simulink library "arduinodue_drivers"  (R2015a)
settings: Solver=ode45  StartTime=0.0  StopTime=10.0  FixedStep=0.01  RelTol=1e-3
settings Model: CovSFcnEnable=off  Creator=odufour  LastModifiedBy=tbaroche
settings DataIOCC: LimitDataPoints=off  SignalLoggingSaveFormat=ModelDataLogs  SignalLogging=off  DSMLogging=off
settings DebuggingCC: UnderspecifiedInitializationDetection=Classic  MergeDetectMultiDrivingBlocksExec=none  SolverPrmCheckMsg=warning
settings GRTTargetCC: CombineOutputUpdateFcns=off  GRTInterface=on

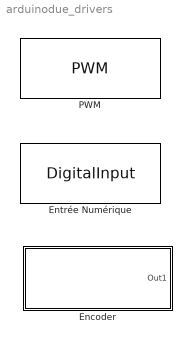
== system arduinodue_drivers ==
  Encoder : Subsystem  mask{pinA=18, pinB=19}
      mask prompts: pinA "Pin A"; pinB "Pin B"
      mask help:
      | Se bloc permet de récupérer le nombre d'incrément qui ont été effectué depuis le lancement de la simulation. Les changements de sens de rotation éventuels sont pris en compte. Ceci permet alors de pouvoir estimer la distance parcourrue.
      |
      | Il est nécessaire d'indiquer les deux entrées sur lesquels est connecté l'encodeur.
      mask Display: disp('Arduino Encoder')
  Entrée Numérique : S-Function  FunctionName=DigitalInput  Parameters=pinNumber, isPullUp  mask(Arduino Digital Input){pinNumber=0, isPullUp=on}
      mask prompts: pinNumber "Pin Number"; isPullUp "Enable Pull Up"
      mask help:
      | Get the logical value of a specified digital input pin.
      |
      | Enter the number of the digital input pin (0-53 for Arduino Due). Do not assign the same pin number to multiple blocks within a model.
      mask init:
      | % Make sure that data type of pinNumber is UINT8
      | pinNumber = uint8(pinNumber);
      | 
      | % Make sure that data type of isPullUp is UINT8
      | isPullUp = uint8(isPullUp);
      mask Display: disp(sprintf('Arduino Digital Input\nPin n°%d',pinNumber))
  PWM : S-Function  FunctionName=PWM  Parameters=pinNumber  mask(Arduino PWM){pinNumber=2}
      mask prompts: pinNumber "Pin Number"
      mask help:
      | Generate square waveform on the specified analog output pin. The block input controls the duty cycle of the square waveform. An input value of 0 produces a 0 percent duty cycle, and an input value of 255 produces a 100 percent duty cycle. The frequency of the waveform is constant at approximately 490 Hz.
      |
      | Enter the number of the analog output pin (2-13 for Arduino Due). Do not assign the same pin number to multiple blocks within a model.
      mask init:
      | % Make sure that pinNumber is an INT32
      | pinNumber = int32(pinNumber);
      mask Display: disp(sprintf('Arduino PWM\nPin n°%d',pinNumber))

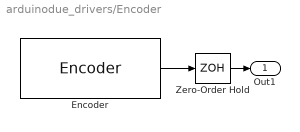
== system arduinodue_drivers/Encoder ==
  Encoder : S-Function  FunctionName=Encoder  Parameters=pinA,pinB  mask(Arduino Encoder){pinA=pinA, pinB=pinB}
      mask prompts: pinA "Pin A"; pinB "Pin B"
      mask init:
      | pinA = uint8(pinA);
      | pinB = uint8(pinB);
      mask Display: disp('Arduino Encoder')
  Zero-Order Hold : ZeroOrderHold  SampleTime=-1
  Out1 : Outport
  wires:
  Zero-Order Hold/1 -> Out1/1
  Encoder/1 -> Zero-Order Hold/1
